simulink model "power_13NodeTestFeeder_4VSC_PV_DEG_symmtrc_loads_"  (R2024b)
settings: Solver=ode15s  StartTime=0.0  StopTime=5  FixedStep=1e-6  MaxStep=1e-4  RelTol=1e-6  AbsTol=1e-8  EnableMultiTasking=on
PreLoadFcn:
  | %power_13NodeTestFeeder_init;
values from neighbouring files (symbols this model uses):
  a = 1.3    [init_para_with_symmtrc_loads.m]
  Cdc = 278e-3    (= 0.278)    [init_para_with_symmtrc_loads.m]
  fg = 60    [a01_scan_VSC_13_feeder.m]    (also in init_para_with_symmtrc_loads.m)
  Gn = 1000    [init_para_with_symmtrc_loads.m]
  H = 8    [init_para_with_symmtrc_loads.m]
  Ipv_n = Isc_n*(Rp+Rs)/Rp    (= 8.21426513558)    [init_para_with_symmtrc_loads.m]
  Isc_n = 8.21    [init_para_with_symmtrc_loads.m]
  k = 1.3806503e-23    [init_para_with_symmtrc_loads.m]    (also in ypm_plot_compare_ana_meas.m = 2)
  Kdroop = Sn/(Rdroop*60)    (= 4166666.66667)    [init_para_with_symmtrc_loads.m]
  KI = 0.0032    [init_para_with_symmtrc_loads.m]
  Ki_C = Rc/tau_C    (= 0.768)    [init_para_with_symmtrc_loads.m]
  Ki_DC = omega_DC^2*Cdc    [init_para_with_symmtrc_loads.m]
  ki_dvpp = kp_dvpp/Ti_dvpp    [init_para_with_symmtrc_loads.m]
  Ki_P = 1/(Ki_pq*tau_P)    [init_para_with_symmtrc_loads.m]
  Ki_PLL = Kp_PLL/tau_PLL    [init_para_with_symmtrc_loads.m]
  Kp_C = Lc/tau_C    (= 0.020372)    [init_para_with_symmtrc_loads.m]
  Kp_DC = 2*xi_DC*omega_DC*Cdc    [init_para_with_symmtrc_loads.m]
  kp_dvpp = -(2*Kdcgain)^-1    [init_para_with_symmtrc_loads.m]
  Kp_P = tau_C/(Ki_pq*tau_P)    [init_para_with_symmtrc_loads.m]
  Kp_PLL = xi_PLL*2*omega_PLL/Vp    [init_para_with_symmtrc_loads.m]
  KV = -0.123    [init_para_with_symmtrc_loads.m]
  kv_Vp = [ 1.021 1.042 1.0174]    [init_para_with_symmtrc_loads.m]
  KVmp = Vmp_n/Voc_n    (= 0.799392097264)    [init_para_with_symmtrc_loads.m]
  Lc = 20.372e-6    (= 2.0372e-05)    [init_para_with_symmtrc_loads.m]
  Lg = Xg /(2*pi*fg)    [init_para_with_symmtrc_loads.m]
  Np = 345    [init_para_with_symmtrc_loads.m]
  Ns = 45    [init_para_with_symmtrc_loads.m]
  Ns_cell = 54    [init_para_with_symmtrc_loads.m]
  p_jump_time = 5    [init_para_with_symmtrc_loads.m]
  p_jump_value = 2*-1e6    (= -2000000)    [init_para_with_symmtrc_loads.m]
  phi_vec = phi_vec_deg/180*pi    [init_para_with_symmtrc_loads.m]
  ppv_nom = 4.9687e+05    (= 496870)    [init_para_with_symmtrc_loads.m]
  q = 1.6021764e-19    [init_para_with_symmtrc_loads.m]
  Rc = 0.768e-3    (= 0.000768)    [init_para_with_symmtrc_loads.m]
  Rg = (U_rms^2 / S_sc) / (sqrt(1 + XoverR^2))    [init_para_with_symmtrc_loads.m]
  Rp = 425.405    [init_para_with_symmtrc_loads.m]
  Rs = 0.221    [init_para_with_symmtrc_loads.m]
  S_base_all = 1    [init_para_with_symmtrc_loads.m]
  Sn = 15e6    (= 15000000)    [init_para_with_symmtrc_loads.m]
  tau_PLL = 2*xi_PLL/omega_PLL    [init_para_with_symmtrc_loads.m]
  Tn = 25    [init_para_with_symmtrc_loads.m]
  Ts = T_ctrl/n_ctrl    [a01_scan_VSC_13_feeder.m]    (also in init_para_with_symmtrc_loads.m = 5e-05)
  U_rms = 4160    [init_para_with_symmtrc_loads.m]
  Vdc = 1200    [init_para_with_symmtrc_loads.m]
  Voc_n = 32.9    [init_para_with_symmtrc_loads.m]
  Vp = sqrt(2)*480/sqrt(3)    [a01_scan_VSC_13_feeder.m]    (also in init_para_with_symmtrc_loads.m = Ug*sqrt(2)/sqrt(3))
undefined symbols (not defined in the file or in its folder): j, Newton, para_grid, para_PVgeno, Raphson
libraries: spsabctoAlphaBetaZeroLib x141, spsPower3phInstantaneousLib x70, spsSeriesRLCBranchLib x44, spsThreePhaseVIMeasurementLib x27, slpidlib x24, spsThreePhaseSeriesRLCLoadLib x15, spsControlledVoltageSourceLib x15, spsMeanLib x9, spsCurrentMeasurementLib x8, spsControlledCurrentSourceLib x8, cstblocks x8, spsGroundLib x5
(part 10 of 10)

== system power_13NodeTestFeeder_4VSC_PV_DEG_symmtrc_loads_/RMS and Pos // Neg Sequence Calculation /Subsystem2/PLL aligned with positive-sequence/Subsystem ==
  note: PI controller with reset port and initial conditions restored after reset or after maximum/minimum values are reached
  in : Inport
  Reset : Inport  Port=2
  Compare To Constant2 : simulink/Logic and Bit Operations/Compare To Constant  relop=~=  const=0  OutDataTypeStr=boolean
  Constant2 : Constant  Value=2*pi*fg
  Gain : Gain  Gain=Kp_PLL
  Gain1 : Gain  Gain=Kp_PLL/tau_PLL
  Integrator Limited : Integrator  ExternalReset=level  InitialCondition=2*pi*fg  UpperSaturationLimit=10.1*2*pi*fg  LowerSaturationLimit=0.09*2*pi*fg  ShowSaturationPort=on
  Memory1 : Memory
  NOT : Logic  Operator=NOT  IconShape=distinctive  AllPortsSameDT=off  OutDataTypeStr=boolean
  OR2 : Logic  Operator=OR  IconShape=distinctive  AllPortsSameDT=off  OutDataTypeStr=boolean
  Product : Product
  Sum : Sum
  Switch1 : Switch  SaturateOnIntegerOverflow=off  InputSameDT=off
  w : Outport
  wires:
  Switch1/1 -> w/1
  Product/1 -> Gain1/1, Gain/1
  Gain1/1 -> Integrator Limited/1
  Integrator Limited/2 -> Compare To Constant2/1, Switch1/2
  Compare To Constant2/1 -> Memory1/1
  OR2/1 -> Integrator Limited/2, NOT/1
  Constant2/1 -> Switch1/3
  Memory1/1 -> OR2/1
  Reset/1 -> OR2/2
  Gain/1 -> Sum/1
  Integrator Limited/1 -> Sum/2
  Sum/1 -> Switch1/1
  in/1 -> Product/1
  NOT/1 -> Product/2

== system power_13NodeTestFeeder_4VSC_PV_DEG_symmtrc_loads_/PV_Geno_GFL_VSC_at_634/PV-Geno with VSC_GFL_at_634     /VSC Control/Current Control/Inverse Park Transformation ==
  qd0 : Inport
  theta : Inport  Port=2
  Constant2 : Constant
  Constant3 : Constant  Value=2*pi/3
  Cos : Trigonometry  Operator=cos
  Matrix Concatenate : Concatenate  NumInputs=3  Mode=Multidimensional array  ConcatenateDimension=2
  Matrix Multiply : Product  Multiplication=Matrix(*)
  Mux1 : Mux  Inputs=3
  Mux2 : Mux  Inputs=3
  Sin : Trigonometry
  Sum : Sum  Inputs=+-|
  Sum1 : Sum  Inputs=++|
  abc : Outport
  wires:
  Constant3/1 -> Sum/2, Sum1/2
  theta/1 -> Mux1/1, Sum1/1, Sum/1
  qd0/1 -> Matrix Multiply/2
  Sum/1 -> Mux1/2
  Sum1/1 -> Mux1/3
  Matrix Multiply/1 -> abc/1
  Mux2/1 -> Matrix Concatenate/3
  Matrix Concatenate/1 -> Matrix Multiply/1
  Mux1/1 -> Cos/1, Sin/1
  Cos/1 -> Matrix Concatenate/1
  Constant2/1 -> Mux2/2, Mux2/3, Mux2/1
  Sin/1 -> Matrix Concatenate/2

== system power_13NodeTestFeeder_4VSC_PV_DEG_symmtrc_loads_/PV_Geno_GFL_VSC_at_634/PV-Geno with VSC_GFL_at_634     /VSC Control/PLL/Park Transformation ==
  abc : Inport
  theta : Inport  Port=2
  Constant3 : Constant  Value=1/2
  Constant5 : Constant  Value=2*pi/3
  Cos : Trigonometry  Operator=cos
  Cos1 : Trigonometry  Operator=cos
  Cos2 : Trigonometry  Operator=cos
  Gain : Gain  Gain=2/3
  Matrix Concatenate : Concatenate  NumInputs=3  Mode=Multidimensional array  ConcatenateDimension=2
  Matrix Multiply : Product  Multiplication=Matrix(*)
  Mux1 : Mux  Inputs=3
  Mux2 : Mux  Inputs=3
  Mux3 : Mux  Inputs=3
  Sin : Trigonometry
  Sin1 : Trigonometry
  Sin2 : Trigonometry
  Sum : Sum  Inputs=+-|
  Sum1 : Sum  Inputs=++|
  qd0 : Outport
  wires:
  Constant5/1 -> Sum1/2, Sum/2
  Matrix Multiply/1 -> qd0/1
  Matrix Concatenate/1 -> Gain/1
  Sin1/1 -> Mux2/2
  Mux3/1 -> Matrix Concatenate/3
  Cos1/1 -> Mux2/1
  Mux1/1 -> Matrix Concatenate/1
  Cos2/1 -> Mux3/1
  Sum/1 -> Cos1/1, Sin1/1
  Mux2/1 -> Matrix Concatenate/2
  Sin/1 -> Mux1/2
  Sin2/1 -> Mux3/2
  Constant3/1 -> Mux1/3, Mux2/3, Mux3/3
  theta/1 -> Sin/1, Cos/1, Sum/1, Sum1/1
  Gain/1 -> Matrix Multiply/1
  Cos/1 -> Mux1/1
  abc/1 -> Matrix Multiply/2
  Sum1/1 -> Cos2/1, Sin2/1

== system power_13NodeTestFeeder_4VSC_PV_DEG_symmtrc_loads_/PV_Geno_GFL_VSC_at_672/PV-Geno with VSC_GFL_at_672/VSC Control/Current Control/Inverse Park Transformation ==
  qd0 : Inport
  theta : Inport  Port=2
  Constant2 : Constant
  Constant3 : Constant  Value=2*pi/3
  Cos : Trigonometry  Operator=cos
  Matrix Concatenate : Concatenate  NumInputs=3  Mode=Multidimensional array  ConcatenateDimension=2
  Matrix Multiply : Product  Multiplication=Matrix(*)
  Mux1 : Mux  Inputs=3
  Mux2 : Mux  Inputs=3
  Sin : Trigonometry
  Sum : Sum  Inputs=+-|
  Sum1 : Sum  Inputs=++|
  abc : Outport
  wires:
  Constant3/1 -> Sum/2, Sum1/2
  theta/1 -> Mux1/1, Sum1/1, Sum/1
  qd0/1 -> Matrix Multiply/2
  Sum/1 -> Mux1/2
  Sum1/1 -> Mux1/3
  Matrix Multiply/1 -> abc/1
  Mux2/1 -> Matrix Concatenate/3
  Matrix Concatenate/1 -> Matrix Multiply/1
  Mux1/1 -> Cos/1, Sin/1
  Cos/1 -> Matrix Concatenate/1
  Constant2/1 -> Mux2/2, Mux2/3, Mux2/1
  Sin/1 -> Matrix Concatenate/2

== system power_13NodeTestFeeder_4VSC_PV_DEG_symmtrc_loads_/PV_Geno_GFL_VSC_at_672/PV-Geno with VSC_GFL_at_672/VSC Control/PLL/Park Transformation ==
  abc : Inport
  theta : Inport  Port=2
  Constant3 : Constant  Value=1/2
  Constant5 : Constant  Value=2*pi/3
  Cos : Trigonometry  Operator=cos
  Cos1 : Trigonometry  Operator=cos
  Cos2 : Trigonometry  Operator=cos
  Gain : Gain  Gain=2/3
  Matrix Concatenate : Concatenate  NumInputs=3  Mode=Multidimensional array  ConcatenateDimension=2
  Matrix Multiply : Product  Multiplication=Matrix(*)
  Mux1 : Mux  Inputs=3
  Mux2 : Mux  Inputs=3
  Mux3 : Mux  Inputs=3
  Sin : Trigonometry
  Sin1 : Trigonometry
  Sin2 : Trigonometry
  Sum : Sum  Inputs=+-|
  Sum1 : Sum  Inputs=++|
  qd0 : Outport
  wires:
  Constant5/1 -> Sum1/2, Sum/2
  Matrix Multiply/1 -> qd0/1
  Matrix Concatenate/1 -> Gain/1
  Sin1/1 -> Mux2/2
  Mux3/1 -> Matrix Concatenate/3
  Cos1/1 -> Mux2/1
  Mux1/1 -> Matrix Concatenate/1
  Cos2/1 -> Mux3/1
  Sum/1 -> Cos1/1, Sin1/1
  Mux2/1 -> Matrix Concatenate/2
  Sin/1 -> Mux1/2
  Sin2/1 -> Mux3/2
  Constant3/1 -> Mux1/3, Mux2/3, Mux3/3
  theta/1 -> Sin/1, Cos/1, Sum/1, Sum1/1
  Gain/1 -> Matrix Multiply/1
  Cos/1 -> Mux1/1
  abc/1 -> Matrix Multiply/2
  Sum1/1 -> Cos2/1, Sin2/1

== system power_13NodeTestFeeder_4VSC_PV_DEG_symmtrc_loads_/PV_Geno_GFL_VSC_at_675/PV-Geno with VSC_GFL_at_675/VSC Control/Current Control/Inverse Park Transformation ==
  qd0 : Inport
  theta : Inport  Port=2
  Constant2 : Constant
  Constant3 : Constant  Value=2*pi/3
  Cos : Trigonometry  Operator=cos
  Matrix Concatenate : Concatenate  NumInputs=3  Mode=Multidimensional array  ConcatenateDimension=2
  Matrix Multiply : Product  Multiplication=Matrix(*)
  Mux1 : Mux  Inputs=3
  Mux2 : Mux  Inputs=3
  Sin : Trigonometry
  Sum : Sum  Inputs=+-|
  Sum1 : Sum  Inputs=++|
  abc : Outport
  wires:
  Constant3/1 -> Sum/2, Sum1/2
  theta/1 -> Mux1/1, Sum1/1, Sum/1
  qd0/1 -> Matrix Multiply/2
  Sum/1 -> Mux1/2
  Sum1/1 -> Mux1/3
  Matrix Multiply/1 -> abc/1
  Mux2/1 -> Matrix Concatenate/3
  Matrix Concatenate/1 -> Matrix Multiply/1
  Mux1/1 -> Cos/1, Sin/1
  Cos/1 -> Matrix Concatenate/1
  Constant2/1 -> Mux2/2, Mux2/3, Mux2/1
  Sin/1 -> Matrix Concatenate/2

== system power_13NodeTestFeeder_4VSC_PV_DEG_symmtrc_loads_/PV_Geno_GFL_VSC_at_675/PV-Geno with VSC_GFL_at_675/VSC Control/PLL/Park Transformation ==
  abc : Inport
  theta : Inport  Port=2
  Constant3 : Constant  Value=1/2
  Constant5 : Constant  Value=2*pi/3
  Cos : Trigonometry  Operator=cos
  Cos1 : Trigonometry  Operator=cos
  Cos2 : Trigonometry  Operator=cos
  Gain : Gain  Gain=2/3
  Matrix Concatenate : Concatenate  NumInputs=3  Mode=Multidimensional array  ConcatenateDimension=2
  Matrix Multiply : Product  Multiplication=Matrix(*)
  Mux1 : Mux  Inputs=3
  Mux2 : Mux  Inputs=3
  Mux3 : Mux  Inputs=3
  Sin : Trigonometry
  Sin1 : Trigonometry
  Sin2 : Trigonometry
  Sum : Sum  Inputs=+-|
  Sum1 : Sum  Inputs=++|
  qd0 : Outport
  wires:
  Constant5/1 -> Sum1/2, Sum/2
  Matrix Multiply/1 -> qd0/1
  Matrix Concatenate/1 -> Gain/1
  Sin1/1 -> Mux2/2
  Mux3/1 -> Matrix Concatenate/3
  Cos1/1 -> Mux2/1
  Mux1/1 -> Matrix Concatenate/1
  Cos2/1 -> Mux3/1
  Sum/1 -> Cos1/1, Sin1/1
  Mux2/1 -> Matrix Concatenate/2
  Sin/1 -> Mux1/2
  Sin2/1 -> Mux3/2
  Constant3/1 -> Mux1/3, Mux2/3, Mux3/3
  theta/1 -> Sin/1, Cos/1, Sum/1, Sum1/1
  Gain/1 -> Matrix Multiply/1
  Cos/1 -> Mux1/1
  abc/1 -> Matrix Multiply/2
  Sum1/1 -> Cos2/1, Sin2/1

== system power_13NodeTestFeeder_4VSC_PV_DEG_symmtrc_loads_/PV_Geno_GFL_VSC_at_680/PV-Geno with VSC_GFL_at_680/VSC Control/Current Control/Inverse Park Transformation ==
  qd0 : Inport
  theta : Inport  Port=2
  Constant2 : Constant
  Constant3 : Constant  Value=2*pi/3
  Cos : Trigonometry  Operator=cos
  Matrix Concatenate : Concatenate  NumInputs=3  Mode=Multidimensional array  ConcatenateDimension=2
  Matrix Multiply : Product  Multiplication=Matrix(*)
  Mux1 : Mux  Inputs=3
  Mux2 : Mux  Inputs=3
  Sin : Trigonometry
  Sum : Sum  Inputs=+-|
  Sum1 : Sum  Inputs=++|
  abc : Outport
  wires:
  Sin/1 -> Matrix Concatenate/2
  Constant2/1 -> Mux2/1, Mux2/3, Mux2/2
  Cos/1 -> Matrix Concatenate/1
  Mux1/1 -> Sin/1, Cos/1
  Matrix Concatenate/1 -> Matrix Multiply/1
  Mux2/1 -> Matrix Concatenate/3
  Matrix Multiply/1 -> abc/1
  Sum1/1 -> Mux1/3
  Sum/1 -> Mux1/2
  qd0/1 -> Matrix Multiply/2
  theta/1 -> Sum/1, Sum1/1, Mux1/1
  Constant3/1 -> Sum1/2, Sum/2

== system power_13NodeTestFeeder_4VSC_PV_DEG_symmtrc_loads_/PV_Geno_GFL_VSC_at_680/PV-Geno with VSC_GFL_at_680/VSC Control/PLL/Park Transformation ==
  abc : Inport
  theta : Inport  Port=2
  Constant3 : Constant  Value=1/2
  Constant5 : Constant  Value=2*pi/3
  Cos : Trigonometry  Operator=cos
  Cos1 : Trigonometry  Operator=cos
  Cos2 : Trigonometry  Operator=cos
  Gain : Gain  Gain=2/3
  Matrix Concatenate : Concatenate  NumInputs=3  Mode=Multidimensional array  ConcatenateDimension=2
  Matrix Multiply : Product  Multiplication=Matrix(*)
  Mux1 : Mux  Inputs=3
  Mux2 : Mux  Inputs=3
  Mux3 : Mux  Inputs=3
  Sin : Trigonometry
  Sin1 : Trigonometry
  Sin2 : Trigonometry
  Sum : Sum  Inputs=+-|
  Sum1 : Sum  Inputs=++|
  qd0 : Outport
  wires:
  Sum1/1 -> Sin2/1, Cos2/1
  abc/1 -> Matrix Multiply/2
  Cos/1 -> Mux1/1
  Gain/1 -> Matrix Multiply/1
  theta/1 -> Sum1/1, Sum/1, Cos/1, Sin/1
  Constant3/1 -> Mux3/3, Mux2/3, Mux1/3
  Sin2/1 -> Mux3/2
  Sin/1 -> Mux1/2
  Mux2/1 -> Matrix Concatenate/2
  Sum/1 -> Sin1/1, Cos1/1
  Cos2/1 -> Mux3/1
  Mux1/1 -> Matrix Concatenate/1
  Cos1/1 -> Mux2/1
  Mux3/1 -> Matrix Concatenate/3
  Sin1/1 -> Mux2/2
  Matrix Concatenate/1 -> Gain/1
  Matrix Multiply/1 -> qd0/1
  Constant5/1 -> Sum/2, Sum1/2

== matlab function power_13NodeTestFeeder_4VSC_PV_DEG_symmtrc_loads_/Dyn_Equivalent of Extended Grid 4.160 kV/Three-phase system ==
  data: fg input; v output; U_rms input; t input
function v = fcn(fg,U_rms,t)

kv_Vp = [ 1 1 1];   % V peak asymmetric gain factors 
                                 % see 13 feeder grid 

Vp = U_rms / sqrt(3) * sqrt(2);

va = Vp * kv_Vp(1) * sin(2*pi*fg*t);
vb = Vp * kv_Vp(2) * sin(2*pi*fg*t - 2*pi/3);
vc = Vp * kv_Vp(3) * sin(2*pi*fg*t + 2*pi/3);

v = [va, vb, vc].';
